simulink model "P_decouple_single_rov"  (Simulink 6.0)
settings: Solver=ode45  StartTime=0.0  StopTime=650  RelTol=1e-3
undefined symbols (not defined in the file): B, DQ, DQL, I, m, M, Ma, MaU, rg, sigbuilder_block, T, W, xb, xg, Xudot, yb, yg, Yvdot, zb, zg, Zwdot
libraries: simulink_extras x8, simulink x7
(part 1 of 2)
settings Model: LastModifiedBy=c chin

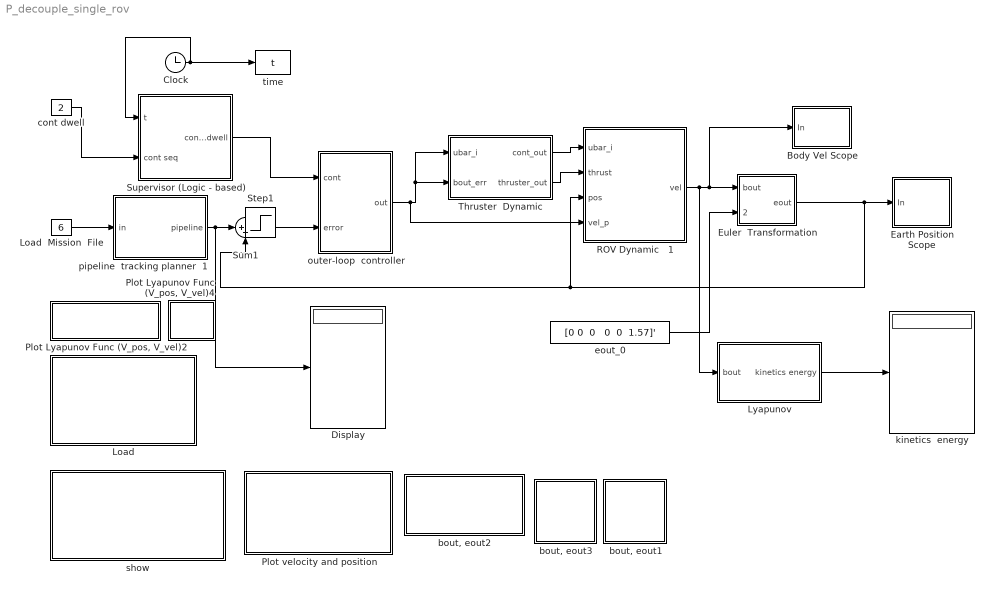
== system P_decouple_single_rov ==
  " Load  " : Subsystem  AncestorBlock=|
      | rov_design_analysis/ROV Controller
      | Design
      | Applications/ Load RRCROV2 parameters
      settings: OpenFcn=|
      | clc
      | cd c:\Matlab7\toolbox\rov_design_analysis\\mat_file ;
      | load rrcrovf;
      mask Display: disp('Double-click \n to \n Load the\n RRCROV\n parameters')
  " ROV Dynamic   1" : Subsystem
      mask Display:
      | disp('ROV')
      | image(imread('/rov_design_analysis/fig/ROVRRC2.jpg'));
      | color('white');port_label('input',1,'ubar_i')
      | color('white');port_label('input',2,'thrust')
      | color('white');port_label('input',3,'eout')
      | color('white');port_label('input',4,'bout_p')
      | 
      | color('white');port_label('output',1,'vel')
  Body Vel Scope : Subsystem  AncestorBlock=|
      | rov_design_analysis/ROV Controller
      | Design
      | Applications/1. Heading autopilot/Earth Position
      | Scope
      mask Display: disp('Body\nVelocity\nScope')
  Clock : Clock
      settings: Decimation=10
  Display : Display
  "Earth Position Scope " : Subsystem  AncestorBlock=|
      | rov_design_analysis/ROV Controller
      | Design
      | Applications/1. Heading autopilot/Earth Position
      | Scope
      mask Display: disp('Earth\nPosition\nScope')
  Euler  Transformation : Subsystem  AncestorBlock=rov_design_analysis/Scope Utilities/Euler Transformation
      mask Display: disp('Navigation \n Sensor')
  Load  Mission  File : Constant  Value=6
  Lyapunov : Subsystem  AncestorBlock=|
      | rov_design_analysis/ROV Controller
      | Design
      | Applications/1. Heading autopilot/pipe tracking
      | profile
      | (Auto)
  "Plot Lyapunov Func (V_pos, V_vel)2" : Subsystem  AncestorBlock=|
      | rov_design_analysis/ROV Controller
      | Design
      | Applications/Plot velocity and position
      settings: OpenFcn=|
      | clc
      | close all
      mask Display: disp('Close All Figure')
  "Plot Lyapunov Func (V_pos, V_vel)4" : Subsystem  AncestorBlock=|
      | rov_design_analysis/ROV Controller
      | Design
      | Applications/Plot velocity and position
      settings: OpenFcn=|
      | clc
      | clear
      mask Display: disp('Clear')
  Plot velocity and position : Subsystem  AncestorBlock=|
      | rov_design_analysis/ROV Controller
      | Design
      | Applications/Plot velocity and position
      settings: OpenFcn=|
      | clc
      | cd c:\Matlab7\toolbox\rov_design_analysis\\m_file ;
      | run nonlin_resp6
      mask Display: disp('Double-click \n to \n Plot Velocity \n and \n Position')
  Sum1 : Sum  Inputs=|+-  OutDataTypeMode=double  SaturateOnIntegerOverflow=on
  Supervisor (Logic - based) : Subsystem
      mask Display: disp('Supervisor \n (Logic-based)')
  Thruster  Dynamic : Subsystem
      mask Display: disp('Thruster \n Dynamic')
  "bout, eout1" : Subsystem  AncestorBlock=|
      | rov_design_analysis/ROV Controller
      | Design
      | Applications/Plot velocity and position
      settings: OpenFcn=|
      | clc
      | cd c:\Matlab7\toolbox\rov_design_analysis\\m_file ;
      | figure
      | plot(eout(:,1),-eout(:,3))
      | xlabel('x')
      | ylabel('z')
      mask Display: disp('Plot \n XZ ')
  "bout, eout2" : Subsystem  AncestorBlock=|
      | rov_design_analysis/ROV Controller
      | Design
      | Applications/Plot velocity and position
      settings: OpenFcn=|
      | clc
      | cd c:\Matlab7\toolbox\rov_design_analysis\\m_file ;
      | figure
      | plot3(eout(:,1), eout(:,2),-eout(:,3))
      | xlabel('x')
      | ylabel('y')
      | zlabel('z')
      | grid on
      mask Display: disp('Plot \n 3D Response')
  "bout, eout3" : Subsystem  AncestorBlock=|
      | rov_design_analysis/ROV Controller
      | Design
      | Applications/Plot velocity and position
      settings: OpenFcn=|
      | clc
      | cd c:\Matlab7\toolbox\rov_design_analysis\\m_file ;
      | figure
      | plot(eout(:,1), eout(:,2))
      | xlabel('x')
      | ylabel('y')
      mask Display: disp('Plot \n XY ')
  cont dwell : Constant  Value=2
  eout_0 : Constant  Value="[0 0  0   0  0  1.57]'"  OutDataTypeMode=double
  kinetics  energy : Display
  outer-loop  controller : Subsystem  Description=f(x)  AncestorBlock=|
      | rov_design_analysis/ROV Controller
      | Design
      | Applications/1. Heading autopilot/controller
      mask Display: disp('Outer Loop \n Controller')
  pipeline  tracking planner  1 : Subsystem  AncestorBlock=|
      | rov_design_analysis/ROV Controller
      | Design
      | Applications/1. Heading autopilot/pipe tracking
      | profile
      | (Auto)
      mask Display: disp('Pipeline Tracking \n Planner')
  show : Subsystem  AncestorBlock=|
      | rov_design_analysis/ROV Controller
      | Design
      | Applications/ Load RRCROV2 parameters
      settings: OpenFcn=|
      | clc
      | cd  c:\Matlab7\toolbox\rov_design_analysis\hybrid ;
      | open rrcrov2_para
      mask Display: disp('Double-click \n to \n SHOW\n RRCROV\n parameters')
  time : ToWorkspace  VariableName=t  SampleTime=1  SaveFormat=Array
  Step1 : Step  IOType=siggen  SampleTime=0
  wires:
  " ROV Dynamic   1"/1(vel) -> Euler  Transformation/1(bout), Body Vel Scope/1(In), Lyapunov/1(bout)
  Euler  Transformation/1(eout) -> "Earth Position Scope "/1(In), Sum1/2, " ROV Dynamic   1"/3("pos ")
  Clock/1 -> time/1, Supervisor (Logic - based)/1(t)
  pipeline  tracking planner  1/1(pipeline) -> Sum1/1, Display/1
  Supervisor (Logic - based)/1(cont dwell) -> outer-loop  controller/1(cont)
  cont dwell/1 -> Supervisor (Logic - based)/2(cont seq)
  eout_0/1 -> Euler  Transformation/2(eout_0)
  Sum1/1 -> outer-loop  controller/2(error)
  Load  Mission  File/1 -> pipeline  tracking planner  1/1(in)
  Thruster  Dynamic/1(cont_out) -> " ROV Dynamic   1"/1(ubar_i)
  Thruster  Dynamic/2(thruster_out) -> " ROV Dynamic   1"/2("thrust ")
  Lyapunov/1(kinetics energy) -> kinetics  energy/1
  outer-loop  controller/1(out) -> Thruster  Dynamic/2(bout_err), Thruster  Dynamic/1(ubar_i), " ROV Dynamic   1"/4(vel_p)

== system P_decouple_single_rov/ Load   ==

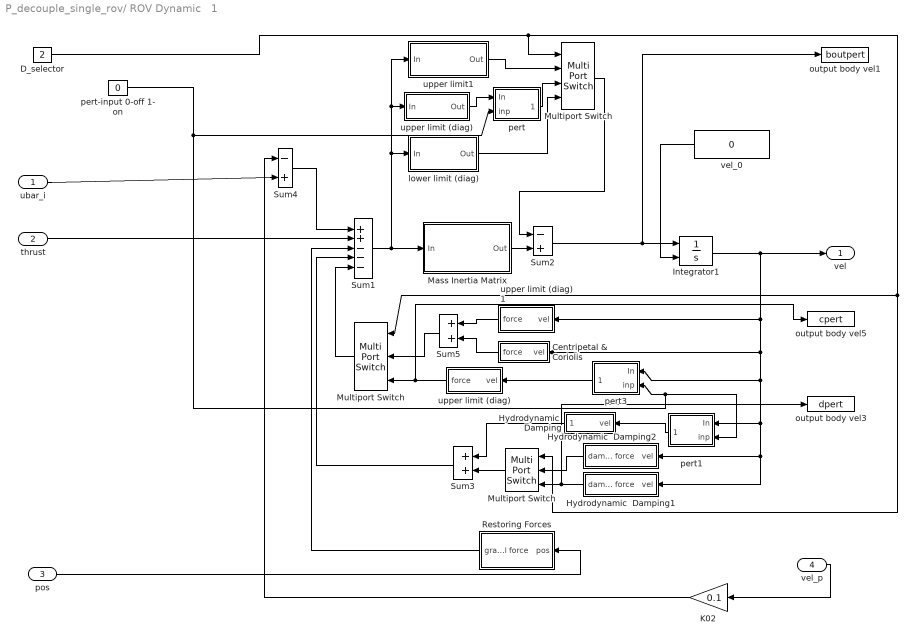
== system P_decouple_single_rov/ ROV Dynamic   1 ==
  ubar_i : Inport  Port=1  LatchInput=off
  "thrust " : Inport  Port=2  LatchInput=off
  "pos " : Inport  Port=3  LatchInput=off
  vel_p : Inport  Port=4  LatchInput=off
  Centripetal & Coriolis : Subsystem  Orientation=left  AncestorBlock=rov_design_analysis/ROV Models/1. Six DOF RRC ROV II/Centripetal & Coriolis
      mask Display: disp('C')
  D_selector : Constant  Value=2
  Hydrodynamic  Damping : Subsystem  Orientation=left
      mask Display: disp('D')
  Hydrodynamic  Damping1 : Subsystem  Orientation=left
      mask Display: disp('perturb \nDamping')
  Hydrodynamic  Damping2 : Subsystem  Orientation=left
      mask Display: disp('Zero Perturb')
  Integrator1 : Integrator  InitialConditionSource=external
  K02 : Gain  Orientation=left  Gain=0.1  SaturateOnIntegerOverflow=on
  Mass Inertia Matrix : Subsystem
      mask Display: disp('inv(MRB+MA)')
  Multiport Switch : MultiPortSwitch  Inputs=3
  "Multiport Switch  " : MultiPortSwitch  Orientation=left  Inputs=2
  "Multiport Switch    " : MultiPortSwitch  Orientation=left  Inputs=2
  Restoring Forces : Subsystem  Orientation=left
      mask Display: disp('Restoring\nForce')
  Sum1 : Sum  Inputs=++---  SaturateOnIntegerOverflow=on  InputSameDT=on
  Sum2 : Sum  Inputs=-+  SaturateOnIntegerOverflow=on  InputSameDT=on
  Sum3 : Sum  Orientation=left  SaturateOnIntegerOverflow=on  InputSameDT=on
  Sum4 : Sum  Inputs=|-+  SaturateOnIntegerOverflow=on  InputSameDT=on
  Sum5 : Sum  Orientation=left  SaturateOnIntegerOverflow=on  InputSameDT=on
  lower limit (diag) : Subsystem
      mask Display: disp('Perturb MA')
  output body vel1 : ToWorkspace  VariableName=boutpert  SampleTime=1  SaveFormat=Array
  output body vel3 : ToWorkspace  VariableName=dpert  SampleTime=1  SaveFormat=Array
  output body vel5 : ToWorkspace  VariableName=cpert  SampleTime=1  SaveFormat=Array
  pert : Subsystem
  pert-input 0-off 1- on : Constant  Value=0
  pert1 : Subsystem  Orientation=left
  pert3 : Subsystem  Orientation=left
  upper limit (diag) : Subsystem
      mask Display: disp('Perturb MA')
  "upper limit (diag)   " : Subsystem  Orientation=left
      mask Display: disp('Perturb CA')
  upper limit (diag)   1 : Subsystem  Orientation=left
      mask Display: disp('CA')
  upper limit1 : Subsystem
      mask Display: disp('Zero Perturb')
  vel_0 : Constant  Orientation=left  Value=0  OutDataTypeMode=double
  vel : Outport
  wires:
  Restoring Forces/1(gravitational force) -> Sum1/3
  "thrust "/1 -> Sum1/2
  Sum1/1 -> Mass Inertia Matrix/1(In), upper limit1/1(In), upper limit (diag)/1(In), lower limit (diag)/1(In)
  "Multiport Switch  "/1 -> Sum1/5
  "pos "/1 -> Restoring Forces/1(pos)
  Mass Inertia Matrix/1(Out) -> Sum2/2
  upper limit1/1(Out) -> Multiport Switch/2
  lower limit (diag)/1(Out) -> Multiport Switch/4
  Multiport Switch/1 -> Sum2/1
  "upper limit (diag)   "/1(force) -> "Multiport Switch  "/3, output body vel5/1
  Sum5/1 -> "Multiport Switch  "/2
  Hydrodynamic  Damping1/1(damping force) -> "Multiport Switch    "/3, output body vel3/1
  Hydrodynamic  Damping2/1(damping force) -> "Multiport Switch    "/2
  Sum3/1 -> Sum1/4
  "Multiport Switch    "/1 -> Sum3/2
  Hydrodynamic  Damping/1(damping force) -> Sum3/1
  upper limit (diag)   1/1(force) -> Sum5/1
  Centripetal & Coriolis/1(force) -> Sum5/2
  Sum2/1 -> output body vel1/1, Integrator1/1
  Integrator1/1 -> vel/1, upper limit (diag)   1/1(vel), Centripetal & Coriolis/1(vel), Hydrodynamic  Damping1/1(vel), Hydrodynamic  Damping2/1(vel), pert1/1(In), pert3/1(In)
  vel_0/1 -> Integrator1/2
  K02/1 -> Sum4/1
  ubar_i/1 -> Sum4/2
  Sum4/1 -> Sum1/1
  vel_p/1 -> K02/1
  pert1/1(on/off) -> Hydrodynamic  Damping/1(vel)
  pert3/1(on/off) -> "upper limit (diag)   "/1(vel)
  upper limit (diag)/1(Out) -> pert/1(In)
  pert/1(on/off) -> Multiport Switch/3
  pert-input 0-off 1- on/1 -> pert/2(inp), pert3/2(inp), pert1/2(inp)
  D_selector/1 -> Multiport Switch/1, "Multiport Switch  "/1, "Multiport Switch    "/1

== system P_decouple_single_rov/Body Vel Scope ==
  In : Inport  Port=1  LatchInput=off
  Demux : Demux  Outputs=6
  output body vel4 : ToWorkspace  VariableName=bout  SampleTime=1  SaveFormat=Array
  phi : Scope
      settings: TickLabels=on  YMin=-0.125  YMax=0.2  DataFormat=Array
  theta : Scope
      settings: TickLabels=on  TimeRange=200  YMin=-0.05  YMax=0.15  DataFormat=Array
  x : Scope
      settings: TickLabels=on  TimeRange=50  YMin=-0.025  YMax=0.375  DataFormat=Array
  y : Scope
      settings: TickLabels=on  YMin=-0.02  YMax=0.1  DataFormat=Array
  yaw : Scope
      settings: TickLabels=on  TimeRange=200  YMin=-0.05  YMax=0.15  SaveName=ScopeData2  DataFormat=Array
  z : Scope
      settings: TickLabels=on  TimeRange=50  YMin=-0.0025  YMax=0.0375  DataFormat=Array
  wires:
  Demux/5 -> theta/1
  In/1 -> Demux/1, output body vel4/1
  Demux/3 -> z/1
  Demux/4 -> phi/1
  Demux/2 -> y/1
  Demux/1 -> x/1
  Demux/6 -> yaw/1

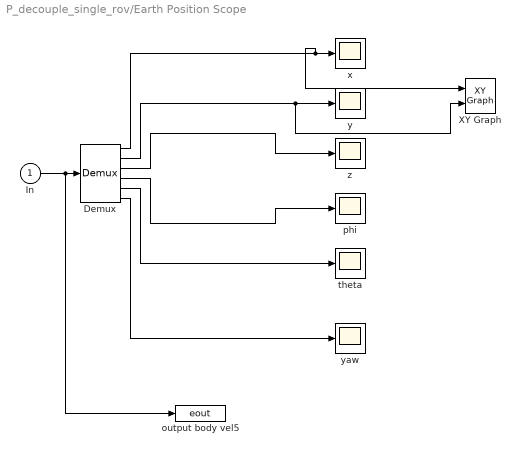
== system P_decouple_single_rov/Earth Position Scope  ==
  In : Inport  Port=1  LatchInput=off
  Demux : Demux  Outputs=6
  XY Graph : simulink/Sinks/XY Graph  xmin=-50  xmax=50  ymin=-50  ymax=50  st=-1
  output body vel5 : ToWorkspace  VariableName=eout  SampleTime=1  SaveFormat=Array
  phi : Scope
      settings: TickLabels=on  YMin=-0.125  YMax=0.2  DataFormat=Array
  theta : Scope
      settings: TickLabels=on  TimeRange=200  YMin=-0.05  YMax=0.15  DataFormat=Array
  x : Scope
      settings: TickLabels=on  TimeRange=50  YMin=-0.025  YMax=0.375  DataFormat=Array
  y : Scope
      settings: TickLabels=on  YMin=-0.02  YMax=0.1  DataFormat=Array
  yaw : Scope
      settings: TickLabels=on  TimeRange=200  YMin=-0.05  YMax=0.15  SaveName=ScopeData2  DataFormat=Array
  z : Scope
      settings: TickLabels=on  TimeRange=50  YMin=-0.0025  YMax=0.0375  DataFormat=Array
  wires:
  Demux/5 -> theta/1
  In/1 -> Demux/1, output body vel5/1
  Demux/3 -> z/1
  Demux/4 -> phi/1
  Demux/2 -> y/1, XY Graph/2
  Demux/1 -> x/1, XY Graph/1
  Demux/6 -> yaw/1

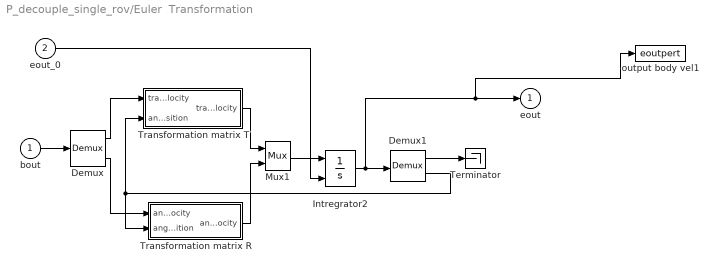
== system P_decouple_single_rov/Euler  Transformation ==
  bout : Inport  Port=1  LatchInput=off
  eout_0 : Inport  Port=2  LatchInput=off
  Demux : Demux  Outputs=2
  Demux1 : Demux  Outputs=2
  Intregrator2 : Integrator  InitialConditionSource=external
  Mux1 : Mux  Inputs=2
  Terminator : Terminator
  Transformation matrix R : Subsystem
      mask Display: disp('Transformation R')
  Transformation matrix T : Subsystem
      mask Display: disp('Transformation T')
  output body vel1 : ToWorkspace  VariableName=eoutpert  SampleTime=1  SaveFormat=Array
  eout : Outport  InitialOutput=0
  wires:
  Mux1/1 -> Intregrator2/1
  Intregrator2/1 -> Demux1/1, eout/1, output body vel1/1
  Demux/2 -> Transformation matrix R/1(angular body  velocity)
  Demux/1 -> Transformation matrix T/1(translational body velocity)
  bout/1 -> Demux/1
  Demux1/2 -> Transformation matrix T/2(angular position), Transformation matrix R/2(angular position)
  Transformation matrix R/1(angular earth velocity) -> Mux1/2
  Transformation matrix T/1(translational earth velocity) -> Mux1/1
  Demux1/1 -> Terminator/1
  eout_0/1 -> Intregrator2/2

== system P_decouple_single_rov/Lyapunov ==
  bout : Inport  Port=1  LatchInput=off
  Gain : Gain  Gain=0.5
  Mass Inertia Matrix1 : Subsystem
      mask Display: disp('MRB+MA')
  Math Function1 : Math  Operator=square  SaturateOnIntegerOverflow=on
  kinetics energy : Outport
  wires:
  Math Function1/1 -> Mass Inertia Matrix1/1(In)
  Gain/1 -> Math Function1/1
  bout/1 -> Gain/1
  Mass Inertia Matrix1/1(Out) -> kinetics energy/1

== system P_decouple_single_rov/Plot Lyapunov Func (V_pos, V_vel)2 ==

== system P_decouple_single_rov/Plot Lyapunov Func (V_pos, V_vel)4 ==

== system P_decouple_single_rov/Plot velocity and position ==

== system P_decouple_single_rov/Supervisor (Logic - based) ==
  t : Inport  Port=1  LatchInput=off
  cont seq : Inport  Port=2  LatchInput=off
  150-300 : Relay  OnSwitchValue=150  OffSwitchValue=0  OnOutputValue=0  OffOutputValue=1
  Constant1 : Constant
  Switching sequence : Subsystem  AncestorBlock=rov_design_analysis/Scope Utilities/Switching sequence
      mask Display: disp('Dwell \n Sequence')
  "cont dwell switch  " : MultiPortSwitch  Inputs=3
  cont dwell : Outport
  wires:
  cont seq/1 -> "cont dwell switch  "/1
  "cont dwell switch  "/1 -> cont dwell/1
  t/1 -> 150-300/1
  Constant1/1 -> "cont dwell switch  "/2
  150-300/1 -> "cont dwell switch  "/3  "1"
  Switching sequence/1(" ") -> "cont dwell switch  "/4  "3"

== system P_decouple_single_rov/Thruster  Dynamic ==
  ubar_i : Inport  Port=1  LatchInput=off
  bout_err : Inport  Port=2  LatchInput=off
  Thruster configuration1 : Subsystem  AncestorBlock=|
      | rov_design_analysis/ROV Controller
      | Design
      | Applications/1. Heading autopilot/Thruster
      | configuration
      mask Display: disp('T')
  Thruster configuration4 : Subsystem  AncestorBlock=|
      | rov_design_analysis/ROV Controller
      | Design
      | Applications/1. Heading autopilot/Thruster
      | configuration
      mask Display: disp('T')
  thruster  dynamic     1 : Subsystem
  thruster  dynamic     2 : Subsystem
  cont_out : Outport
  thruster_out : Outport  Port=2
  wires:
  Thruster configuration1/1(output force) -> thruster_out/1
  thruster  dynamic     1/1(T) -> Thruster configuration4/1(input velocity)
  Thruster configuration4/1(output force) -> cont_out/1
  thruster  dynamic     2/1(T) -> Thruster configuration1/1(input velocity)
  bout_err/1 -> thruster  dynamic     2/1(volt)
  ubar_i/1 -> thruster  dynamic     1/1(volt)

== system P_decouple_single_rov/bout, eout1 ==

== system P_decouple_single_rov/bout, eout2 ==

== system P_decouple_single_rov/bout, eout3 ==

== system P_decouple_single_rov/outer-loop  controller ==
  cont : Inport  Port=1  LatchInput=off
  error : Inport  Port=2  LatchInput=off
  Multiport Switch : MultiPortSwitch  Inputs=2
  "P decoupled " : Subsystem
  PI : Subsystem
  bout input : Constant  Value="[ 0 0  0  0  0 0]'"
  out : Outport
  wires:
  cont/1 -> Multiport Switch/1
  bout input/1 -> "P decoupled "/2(vel_d), "P decoupled "/3(vel)
  Multiport Switch/1 -> out/1
  "P decoupled "/1(" ") -> Multiport Switch/2
  PI/1(" ") -> Multiport Switch/3
  error/1 -> "P decoupled "/1(err), PI/1(err)

== system P_decouple_single_rov/pipeline  tracking planner  1 ==
  in : Inport  Port=1  LatchInput=off
  decoupled input : Subsystem
  pipeline : Outport
  wires:
  in/1 -> decoupled input/1(In1)
  decoupled input/1(Out1) -> pipeline/1

== system P_decouple_single_rov/show ==

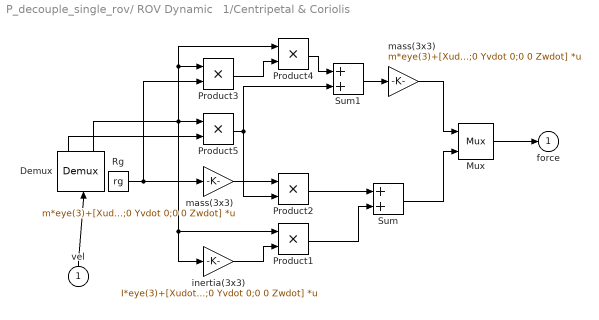
== system P_decouple_single_rov/ ROV Dynamic   1/Centripetal & Coriolis ==
  vel : Inport  Orientation=up  Port=1  LatchInput=off
  Demux : Demux  Orientation=up  Outputs=2
  Mux : Mux  Inputs=2
  Product{1..5} (5 alike) : Product  SaturateOnIntegerOverflow=on  RndMeth=Zero  InputSameDT=on
  Rg : Constant  Value=rg
  Sum : Sum  SaturateOnIntegerOverflow=on  InputSameDT=on
  Sum1 : Sum  SaturateOnIntegerOverflow=on  InputSameDT=on
  inertia(3x3) : Gain  Gain=I*eye(3)+[Xudot 0 0;0 Yvdot 0;0 0 Zwdot]  Multiplication=Matrix(K*u)  SaturateOnIntegerOverflow=on
  "mass(3x3) " : Gain  Gain=m*eye(3)+[Xudot 0 0;0 Yvdot 0;0 0 Zwdot]  Multiplication=Matrix(K*u)  SaturateOnIntegerOverflow=on
  "mass(3x3)   " : Gain  Gain=m*eye(3)+[Xudot 0 0;0 Yvdot 0;0 0 Zwdot]  Multiplication=Matrix(K*u)  SaturateOnIntegerOverflow=on
  force : Outport  InitialOutput=0
  wires:
  Product1/1 -> Sum/2
  "mass(3x3)   "/1 -> Product2/1
  Product2/1 -> Sum/1
  Rg/1 -> Product3/2, "mass(3x3)   "/1
  Product3/1 -> Product4/2
  Product4/1 -> Sum1/1
  Product5/1 -> Product2/2, Sum1/2
  Sum1/1 -> "mass(3x3) "/1
  Demux/2 -> Product5/1, Product3/1, Product4/1, Product1/1, inertia(3x3)/1
  Demux/1 -> Product5/2
  vel/1 -> Demux/1
  inertia(3x3)/1 -> Product1/2
  "mass(3x3) "/1 -> Mux/1
  Sum/1 -> Mux/2
  Mux/1 -> force/1

== system P_decouple_single_rov/ ROV Dynamic   1/Hydrodynamic  Damping ==
  vel : Inport  Port=1  LatchInput=off
  D linear : Gain  Gain=-diag(DQL)  SaturateOnIntegerOverflow=on
  damping force : Outport  InitialOutput=0
  wires:
  vel/1 -> D linear/1
  D linear/1 -> damping force/1

== system P_decouple_single_rov/ ROV Dynamic   1/Hydrodynamic  Damping1 ==
  vel : Inport  Port=1  LatchInput=off
  D quadratic : Gain  Gain=-diag(DQ)  SaturateOnIntegerOverflow=on
  Product : Product  SaturateOnIntegerOverflow=on  RndMeth=Zero  InputSameDT=on
  |u| : Abs  SaturateOnIntegerOverflow=on
  damping force : Outport  InitialOutput=0
  wires:
  Product/1 -> D quadratic/1
  vel/1 -> Product/1, |u|/1
  |u|/1 -> Product/2
  D quadratic/1 -> damping force/1

== system P_decouple_single_rov/ ROV Dynamic   1/Hydrodynamic  Damping2 ==
  vel : Inport  Port=1  LatchInput=off
  D quadratic : Gain  Gain=0  SaturateOnIntegerOverflow=on
  damping force : Outport  InitialOutput=0
  wires:
  vel/1 -> D quadratic/1
  D quadratic/1 -> damping force/1

== system P_decouple_single_rov/ ROV Dynamic   1/Mass Inertia Matrix ==
  In : Inport  Port=1  LatchInput=off
  inverse M : Gain  Gain=inv(M-Ma)  Multiplication=Matrix(K*u)  SaturateOnIntegerOverflow=on
  Out : Outport
  wires:
  inverse M/1 -> Out/1
  In/1 -> inverse M/1

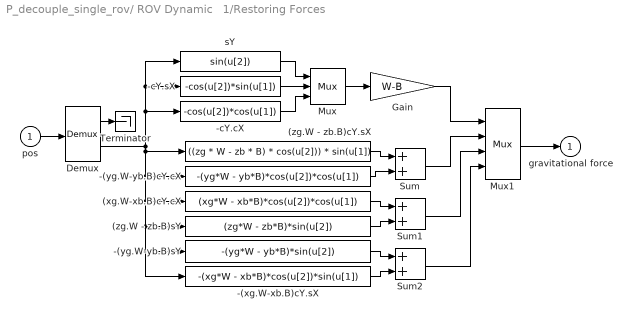
== system P_decouple_single_rov/ ROV Dynamic   1/Restoring Forces ==
  pos : Inport  Port=1  LatchInput=off
  (xg.W-xb.B)cY.cX : Fcn  Expr=(xg*W - xb*B)*cos(u[2])*cos(u[1])
  (zg.W - zb.B)cY.sX : Fcn  Expr=((zg * W - zb * B) * cos(u[2])) * sin(u[1])
  (zg.W - zb.B)sY : Fcn  Expr=(zg*W - zb*B)*sin(u[2])
  -(xg.W-xb.B)cY.sX : Fcn  Expr=-(xg*W - xb*B)*cos(u[2])*sin(u[1])
  -(yg.W-yb.B)cY.cX : Fcn  Expr=-(yg*W - yb*B)*cos(u[2])*cos(u[1])
  -(yg.W-yb.B)sY : Fcn  Expr=-(yg*W - yb*B)*sin(u[2])
  -cY.cX : Fcn  Expr=-cos(u[2])*cos(u[1])
  -cY.sX : Fcn  Expr=-cos(u[2])*sin(u[1])
  Demux : Demux  Outputs=2
  Gain : Gain  Gain=W-B  SaturateOnIntegerOverflow=on
  Mux : Mux  Inputs=3
  Mux1 : Mux
  Sum : Sum  SaturateOnIntegerOverflow=on  InputSameDT=on
  Sum1 : Sum  SaturateOnIntegerOverflow=on  InputSameDT=on
  Sum2 : Sum  SaturateOnIntegerOverflow=on  InputSameDT=on
  Terminator : Terminator
  sY : Fcn  Expr=sin(u[2])
  gravitational force : Outport  InitialOutput=0
  wires:
  Sum2/1 -> Mux1/4
  -(yg.W-yb.B)sY/1 -> Sum2/1
  -(xg.W-xb.B)cY.sX/1 -> Sum2/2
  Sum1/1 -> Mux1/3
  (xg.W-xb.B)cY.cX/1 -> Sum1/1
  (zg.W - zb.B)sY/1 -> Sum1/2
  Sum/1 -> Mux1/2
  (zg.W - zb.B)cY.sX/1 -> Sum/1
  -(yg.W-yb.B)cY.cX/1 -> Sum/2
  Gain/1 -> Mux1/1
  Mux/1 -> Gain/1
  -cY.cX/1 -> Mux/3
  -cY.sX/1 -> Mux/2
  sY/1 -> Mux/1
  Mux1/1 -> gravitational force/1
  Demux/2 -> -(xg.W-xb.B)cY.sX/1, -(yg.W-yb.B)sY/1, (zg.W - zb.B)sY/1, (xg.W-xb.B)cY.cX/1, -(yg.W-yb.B)cY.cX/1, (zg.W - zb.B)cY.sX/1, sY/1, -cY.sX/1, -cY.cX/1
  Demux/1 -> Terminator/1
  pos/1 -> Demux/1

== system P_decouple_single_rov/ ROV Dynamic   1/lower limit (diag) ==
  In : Inport  Port=1  LatchInput=off
  inverse M : Gain  Gain=-diag([21.1403-21.0981 51.7012-51.0026 92.451-91.837 3.6191-3.576 2.6427-2.7687 2.3033-2.3493])  Multiplication=Matrix(K*u)  SaturateOnIntegerOverflow=on
  Out : Outport
  wires:
  inverse M/1 -> Out/1
  In/1 -> inverse M/1

== system P_decouple_single_rov/ ROV Dynamic   1/pert ==
  In : Inport  Port=1  LatchInput=off
  inp : Inport  Port=2  LatchInput=off
  D linear3 : Gain  Gain=2  SaturateOnIntegerOverflow=on
  Product : Product  RndMeth=Zero
  Sine Wave-pert : Sin  Amplitude=0.1  SampleTime=0
  Sum6 : Sum  Inputs=|++  SaturateOnIntegerOverflow=on  InputSameDT=on
  on/off : Outport
  wires:
  D linear3/1 -> Sum6/1
  Sine Wave-pert/1 -> Product/1
  Product/1 -> Sum6/2
  inp/1 -> Product/2
  In/1 -> D linear3/1
  Sum6/1 -> on/off/1

== system P_decouple_single_rov/ ROV Dynamic   1/pert1 ==
  In : Inport  Port=1  LatchInput=off
  inp : Inport  Port=2  LatchInput=off
  D linear3 : Gain  Gain=2  SaturateOnIntegerOverflow=on
  Product : Product  RndMeth=Zero
  Sine Wave-pert : Sin  Amplitude=0.1  SampleTime=0
  Sum6 : Sum  Inputs=|++  SaturateOnIntegerOverflow=on  InputSameDT=on
  on/off : Outport
  wires:
  D linear3/1 -> Sum6/1
  Sine Wave-pert/1 -> Product/1
  Product/1 -> Sum6/2
  inp/1 -> Product/2
  In/1 -> D linear3/1
  Sum6/1 -> on/off/1

== system P_decouple_single_rov/ ROV Dynamic   1/pert3 ==
  In : Inport  Port=1  LatchInput=off
  inp : Inport  Port=2  LatchInput=off
  D linear3 : Gain  Gain=2  SaturateOnIntegerOverflow=on
  Product : Product  RndMeth=Zero
  Sine Wave-pert : Sin  Amplitude=0.1  SampleTime=0
  Sum6 : Sum  Inputs=|++  SaturateOnIntegerOverflow=on  InputSameDT=on
  on/off : Outport
  wires:
  D linear3/1 -> Sum6/1
  Sine Wave-pert/1 -> Product/1
  Product/1 -> Sum6/2
  inp/1 -> Product/2
  In/1 -> D linear3/1
  Sum6/1 -> on/off/1

== system P_decouple_single_rov/ ROV Dynamic   1/upper limit (diag) ==
  In : Inport  Port=1  LatchInput=off
  inverse M : Gain  Gain=-diag([21.724-21.1403 51.7013-51.7012 94.3-92.451 4.2176-3.6191 7.1148-2.6427 4.7673-2.3033])  Multiplication=Matrix(K*u)  SaturateOnIntegerOverflow=on
  Out : Outport
  wires:
  inverse M/1 -> Out/1
  In/1 -> inverse M/1

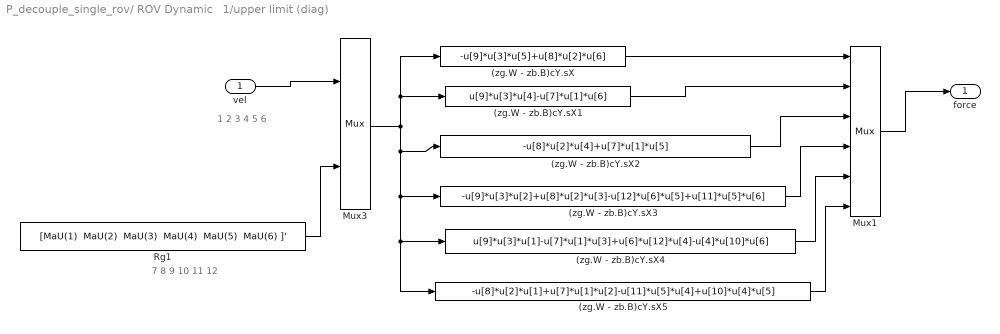
== system P_decouple_single_rov/ ROV Dynamic   1/upper limit (diag)    ==
  note: 7 8 9 10 11 12
  note: 1 2 3 4 5 6
  vel : Inport  Port=1  LatchInput=off
  (zg.W - zb.B)cY.sX : Fcn  Expr=-u[9]*u[3]*u[5]+u[8]*u[2]*u[6]
  (zg.W - zb.B)cY.sX1 : Fcn  Expr=u[9]*u[3]*u[4]-u[7]*u[1]*u[6]
  (zg.W - zb.B)cY.sX2 : Fcn  Expr=-u[8]*u[2]*u[4]+u[7]*u[1]*u[5]
  (zg.W - zb.B)cY.sX3 : Fcn  Expr=-u[9]*u[3]*u[2]+u[8]*u[2]*u[3]-u[12]*u[6]*u[5]+u[11]*u[5]*u[6]
  (zg.W - zb.B)cY.sX4 : Fcn  Expr=u[9]*u[3]*u[1]-u[7]*u[1]*u[3]+u[6]*u[12]*u[4]-u[4]*u[10]*u[6]
  (zg.W - zb.B)cY.sX5 : Fcn  Expr=-u[8]*u[2]*u[1]+u[7]*u[1]*u[2]-u[11]*u[5]*u[4]+u[10]*u[4]*u[5]
  Mux1 : Mux  Inputs=6
  Mux3 : Mux  Inputs=2
  Rg1 : Constant  Value="[MaU(1)  MaU(2)  MaU(3)  MaU(4)  MaU(5)  MaU(6) ]'"
  force : Outport
  wires:
  Mux1/1 -> force/1
  (zg.W - zb.B)cY.sX/1 -> Mux1/1
  (zg.W - zb.B)cY.sX1/1 -> Mux1/2
  (zg.W - zb.B)cY.sX2/1 -> Mux1/3
  (zg.W - zb.B)cY.sX3/1 -> Mux1/4
  (zg.W - zb.B)cY.sX4/1 -> Mux1/5
  (zg.W - zb.B)cY.sX5/1 -> Mux1/6
  vel/1 -> Mux3/1
  Rg1/1 -> Mux3/2
  Mux3/1 -> (zg.W - zb.B)cY.sX/1, (zg.W - zb.B)cY.sX1/1, (zg.W - zb.B)cY.sX4/1, (zg.W - zb.B)cY.sX5/1, (zg.W - zb.B)cY.sX3/1, (zg.W - zb.B)cY.sX2/1

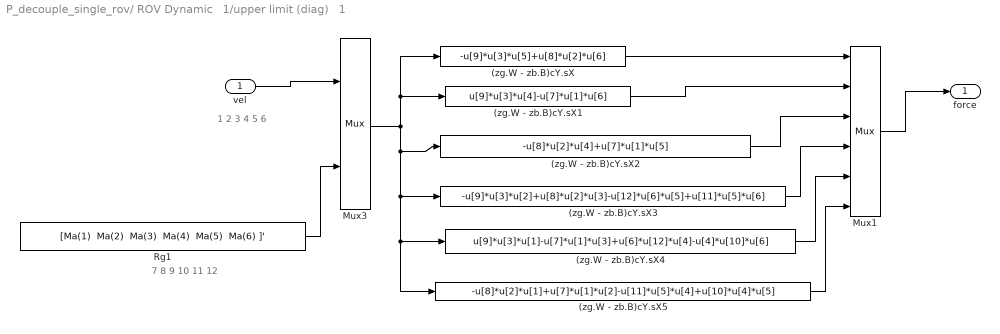
== system P_decouple_single_rov/ ROV Dynamic   1/upper limit (diag)   1 ==
  note: 7 8 9 10 11 12
  note: 1 2 3 4 5 6
  vel : Inport  Port=1  LatchInput=off
  (zg.W - zb.B)cY.sX : Fcn  Expr=-u[9]*u[3]*u[5]+u[8]*u[2]*u[6]
  (zg.W - zb.B)cY.sX1 : Fcn  Expr=u[9]*u[3]*u[4]-u[7]*u[1]*u[6]
  (zg.W - zb.B)cY.sX2 : Fcn  Expr=-u[8]*u[2]*u[4]+u[7]*u[1]*u[5]
  (zg.W - zb.B)cY.sX3 : Fcn  Expr=-u[9]*u[3]*u[2]+u[8]*u[2]*u[3]-u[12]*u[6]*u[5]+u[11]*u[5]*u[6]
  (zg.W - zb.B)cY.sX4 : Fcn  Expr=u[9]*u[3]*u[1]-u[7]*u[1]*u[3]+u[6]*u[12]*u[4]-u[4]*u[10]*u[6]
  (zg.W - zb.B)cY.sX5 : Fcn  Expr=-u[8]*u[2]*u[1]+u[7]*u[1]*u[2]-u[11]*u[5]*u[4]+u[10]*u[4]*u[5]
  Mux1 : Mux  Inputs=6
  Mux3 : Mux  Inputs=2
  Rg1 : Constant  Value="[Ma(1)  Ma(2)  Ma(3)  Ma(4)  Ma(5)  Ma(6) ]'"
  force : Outport
  wires:
  Mux1/1 -> force/1
  (zg.W - zb.B)cY.sX/1 -> Mux1/1
  (zg.W - zb.B)cY.sX1/1 -> Mux1/2
  (zg.W - zb.B)cY.sX2/1 -> Mux1/3
  (zg.W - zb.B)cY.sX3/1 -> Mux1/4
  (zg.W - zb.B)cY.sX4/1 -> Mux1/5
  (zg.W - zb.B)cY.sX5/1 -> Mux1/6
  vel/1 -> Mux3/1
  Rg1/1 -> Mux3/2
  Mux3/1 -> (zg.W - zb.B)cY.sX/1, (zg.W - zb.B)cY.sX1/1, (zg.W - zb.B)cY.sX4/1, (zg.W - zb.B)cY.sX5/1, (zg.W - zb.B)cY.sX3/1, (zg.W - zb.B)cY.sX2/1

== system P_decouple_single_rov/ ROV Dynamic   1/upper limit1 ==
  In : Inport  Port=1  LatchInput=off
  inverse M : Gain  Gain=0  Multiplication=Matrix(K*u)  SaturateOnIntegerOverflow=on
  Out : Outport
  wires:
  inverse M/1 -> Out/1
  In/1 -> inverse M/1

== system P_decouple_single_rov/Euler  Transformation/Transformation matrix R ==
  angular body  velocity : Inport  Port=1  LatchInput=off
  angular position : Inport  Port=2  LatchInput=off
  Mux : Mux  Inputs=3
  Row1 of T : Subsystem
      mask Display: disp('Row 1')
  Row2 of T : Subsystem
      mask Display: disp('Row 2')
  Row3 of T : Subsystem
      mask Display: disp('Row 3')
  angular earth velocity : Outport
  wires:
  angular position/1 -> Row3 of T/2(angular position), Row1 of T/2(angular position), Row2 of T/2(angular position)
  Mux/1 -> angular earth velocity/1
  Row3 of T/1(angular earth velocity (row 3)) -> Mux/3
  Row2 of T/1(angular earth velocity (row 2)) -> Mux/2
  Row1 of T/1(angular earth velocity (row 1)) -> Mux/1
  angular body  velocity/1 -> Row3 of T/1("angular body velocity "), Row2 of T/1("angular body velocity "), Row1 of T/1(angular body  velocity)

== system P_decouple_single_rov/Euler  Transformation/Transformation matrix T ==
  translational body velocity : Inport  Port=1  LatchInput=off
  angular position : Inport  Port=2  LatchInput=off
  Mux : Mux  Inputs=3
  Row1 of R : Subsystem
      mask Display: disp('Row 1')
  Row2 of R : Subsystem
      mask Display: disp('Row 2')
  Row3 of R : Subsystem
      mask Display: disp('Row 3')
  translational earth velocity : Outport  InitialOutput=0
  wires:
  Mux/1 -> translational earth velocity/1
  Row3 of R/1(translational earth velocity (row 3)) -> Mux/3
  Row2 of R/1(translational earth velocity (row 2)) -> Mux/2
  Row1 of R/1(translational earth velocity (row 1)) -> Mux/1
  angular position/1 -> Row3 of R/2(angular position), Row1 of R/2(angular position), Row2 of R/2(angular position)
  translational body velocity/1 -> Row1 of R/1(translational body velocity), Row2 of R/1(translational body velocity), Row3 of R/1(translational body velocity)

== system P_decouple_single_rov/Lyapunov/Mass Inertia Matrix1 ==
  In : Inport  Port=1  LatchInput=off
  inverse M : Gain  Gain=M-Ma  Multiplication=Matrix(K*u)  SaturateOnIntegerOverflow=on
  Out : Outport
  wires:
  inverse M/1 -> Out/1
  In/1 -> inverse M/1

== system P_decouple_single_rov/Supervisor (Logic - based)/Switching sequence ==
  Add2 : Sum  Inputs=+++++++  OutScaling=2^-10
  Signal Builder2 : Subsystem  Tag=STV Subsys  LoadFcn=sigbuilder_block('load');  StartFcn=sigbuilder_block('start');  StopFcn=sigbuilder_block('stop');  ClipboardFcn=sigbuilder_block('clipboard');  mask(Sigbuilder block){}
      mask help: Sigbuilder GUI
      mask init:
      | if ~strcmp(get_param(bdroot(gcbh),'SimulationStatus'),'stopped') tuvar = sigbuilder_block('maskInit'); end
      settings: CopyFcn=sigbuilder_block('copy');  DeleteFcn=sigbuilder_block('delete');  ModelCloseFcn=sigbuilder_block('modelClose');  PreSaveFcn=sigbuilder_block('preSave');  NameChangeFcn=sigbuilder_block('namechange');  OpenFcn=sigbuilder_block('open',[0 19.5 768 499.5 ]);  CloseFcn=sigbuilder_block('close');
      mask Display: plot(0,0,100,100,[10,10,40,40,10],[80,20,20,80,80],[40,10],[50,50], [40,27,10],[65,72,56],[40,25,25,10],[28,28,43,43]);
  " " : Outport
  wires:
  Add2/1 -> " "/1
  Signal Builder2/7(Signal 7) -> Add2/7
  Signal Builder2/6(Signal 6) -> Add2/6
  Signal Builder2/5(Signal 5) -> Add2/5
  Signal Builder2/4(Signal 4) -> Add2/4
  Signal Builder2/3(Signal 3) -> Add2/3
  Signal Builder2/2(Signal 2) -> Add2/2
  Signal Builder2/1(Signal 1) -> Add2/1

== system P_decouple_single_rov/Thruster  Dynamic/Thruster configuration1 ==
  input velocity : Inport  Orientation=up  Port=1  LatchInput=off
  Thruster Matrix : Gain  Gain=T  Multiplication=Matrix(K*u)  SaturateOnIntegerOverflow=on
  output force : Outport  InitialOutput=0
  wires:
  input velocity/1 -> Thruster Matrix/1
  Thruster Matrix/1 -> output force/1

== system P_decouple_single_rov/Thruster  Dynamic/Thruster configuration4 ==
  input velocity : Inport  Orientation=up  Port=1  LatchInput=off
  Thruster Matrix : Gain  Gain=T  Multiplication=Matrix(K*u)  SaturateOnIntegerOverflow=on
  output force : Outport  InitialOutput=0
  wires:
  input velocity/1 -> Thruster Matrix/1
  Thruster Matrix/1 -> output force/1

== system P_decouple_single_rov/Thruster  Dynamic/thruster  dynamic     1 ==
  volt : Inport  Orientation=down  Port=1  LatchInput=off
  Gain2 : Gain  Gain=0.5  SaturateOnIntegerOverflow=on
  Saturation : Saturate  UpperLimit=70  LowerLimit=-70
  "thruster  alloc. " : Subsystem
  T : Outport
  wires:
  volt/1 -> "thruster  alloc. "/1(err)
  "thruster  alloc. "/1(u) -> Gain2/1
  Saturation/1 -> T/1
  Gain2/1 -> Saturation/1

== system P_decouple_single_rov/Thruster  Dynamic/thruster  dynamic     2 ==
  volt : Inport  Orientation=down  Port=1  LatchInput=off
  Gain2 : Gain  Gain=0.5  SaturateOnIntegerOverflow=on
  Saturation : Saturate  UpperLimit=70  LowerLimit=-70
  "thruster  alloc. " : Subsystem
  T : Outport
  wires:
  volt/1 -> "thruster  alloc. "/1(err)
  "thruster  alloc. "/1(u) -> Gain2/1
  Saturation/1 -> T/1
  Gain2/1 -> Saturation/1

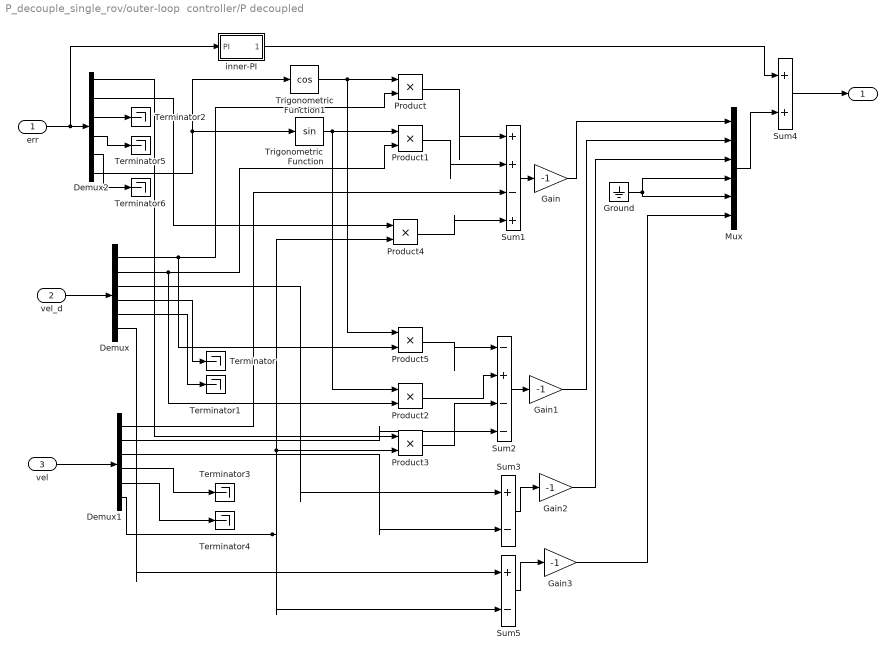
== system P_decouple_single_rov/outer-loop  controller/P decoupled  ==
  err : Inport  Port=1  LatchInput=off
  vel_d : Inport  Port=2  LatchInput=off
  vel : Inport  Port=3  LatchInput=off
  Demux : Demux  Outputs=6
  Demux1 : Demux  Outputs=6
  Demux2 : Demux  Outputs=6
  Gain{,1..3} (4 alike) : Gain  Gain=-1
  Ground : Ground
  Mux : Mux  Inputs=6
  Product{,1..4} (5 alike) : Product  RndMeth=Zero
  Product5 : Product  OutDataTypeMode=double  RndMeth=Zero
  Sum1 : Sum  Inputs=|++-+  SaturateOnIntegerOverflow=on  InputSameDT=on
  Sum2 : Sum  Inputs=|-+--  SaturateOnIntegerOverflow=on  InputSameDT=on
  Sum3 : Sum  Inputs=|+-  SaturateOnIntegerOverflow=on  InputSameDT=on
  Sum4 : Sum  Inputs=|++  SaturateOnIntegerOverflow=on  InputSameDT=on
  Sum5 : Sum  Inputs=|+-  SaturateOnIntegerOverflow=on  InputSameDT=on
  Terminator{,1..6} (7 alike) : Terminator
  Trigonometric Function : Trigonometry
  Trigonometric Function1 : Trigonometry  Operator=cos
  inner-PI : Subsystem
  " " : Outport
  wires:
  err/1 -> Demux2/1, inner-PI/1(PI)
  vel_d/1 -> Demux/1
  Sum2/1 -> Gain1/1
  Sum1/1 -> Gain/1
  Sum3/1 -> Gain2/1
  Ground/1 -> Mux/4, Mux/5
  vel/1 -> Demux1/1
  Demux1/4 -> Terminator3/1
  Demux1/5 -> Terminator4/1
  Trigonometric Function/1 -> Product1/1, Product2/1
  Trigonometric Function1/1 -> Product/1, Product5/1
  Demux2/6 -> Trigonometric Function1/1, Trigonometric Function/1
  Demux/1 -> Product5/2, Product/2
  Demux/2 -> Product2/2, Product1/2
  Product/1 -> Sum1/1
  Product1/1 -> Sum1/2
  Demux1/1 -> Sum1/3
  Product4/1 -> Sum1/4
  Demux1/6 -> Product4/2, Product3/2, Sum5/2
  Demux2/2 -> Product4/1
  Product5/1 -> Sum2/1
  Product2/1 -> Sum2/2
  Product3/1 -> Sum2/3
  Demux2/1 -> Product3/1
  Demux1/2 -> Sum2/4
  Demux/3 -> Sum3/1
  Demux1/3 -> Sum3/2
  Demux/4 -> Terminator/1
  Demux/5 -> Terminator1/1
  Gain/1 -> Mux/1
  Gain1/1 -> Mux/2
  Gain2/1 -> Mux/3
  inner-PI/1(" ") -> Sum4/1
  Mux/1 -> Sum4/2
  Sum4/1 -> " "/1
  Demux2/3 -> Terminator2/1
  Demux2/4 -> Terminator5/1
  Demux2/5 -> Terminator6/1
  Demux/6 -> Sum5/1
  Sum5/1 -> Gain3/1
  Gain3/1 -> Mux/6

== system P_decouple_single_rov/outer-loop  controller/PI ==
  err : Inport  Port=1  LatchInput=off
  Demux1 : Demux  Outputs=6
  Mux2 : Mux  Inputs=6
  P Controller{1..4} (4 alike) : simulink_extras/Additional Linear/PID Controller  P=1  I=1  D=0
  " " : Outport
  wires:
  P Controller3/1 -> Mux2/3
  err/1 -> Demux1/1
  Mux2/1 -> " "/1
  Demux1/1 -> P Controller1/1
  P Controller1/1 -> Mux2/1
  P Controller2/1 -> Mux2/2
  P Controller4/1 -> Mux2/6
  Demux1/2 -> P Controller2/1
  Demux1/3 -> P Controller3/1
  Demux1/6 -> P Controller4/1

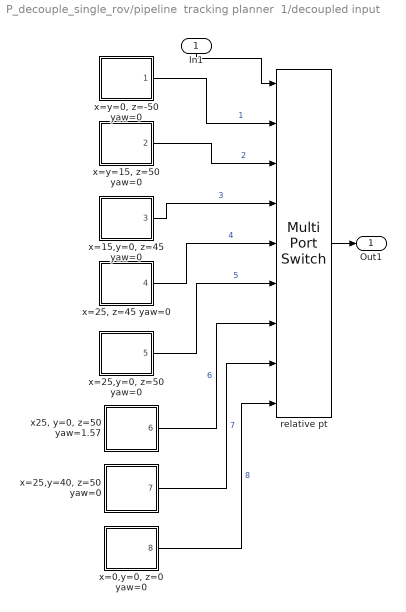
== system P_decouple_single_rov/pipeline  tracking planner  1/decoupled input ==
  In1 : Inport  Orientation=down  Port=1  LatchInput=off
  relative pt : MultiPortSwitch  Inputs=8
  "x25, y=0, z=50 yaw=1.57" : Subsystem
  "x=0,y=0, z=0 yaw=0  " : Subsystem
  "x=15,y=0, z=45 yaw=0 " : Subsystem
  "x=25, z=45 yaw=0" : Subsystem
  "x=25,y=0, z=50 yaw=0" : Subsystem
  "x=25,y=40, z=50 yaw=0" : Subsystem
  "x=y=0, z=-50 yaw=0  " : Subsystem
  "x=y=15, z=50 yaw=0 " : Subsystem
  Out1 : Outport
  wires:
  "x=y=0, z=-50 yaw=0  "/1("1 ") -> relative pt/2  "1"
  "x=y=15, z=50 yaw=0 "/1(2) -> relative pt/3  "2"
  "x=15,y=0, z=45 yaw=0 "/1(3) -> relative pt/4  "3"
  "x=25, z=45 yaw=0"/1(4) -> relative pt/5  "4"
  "x=25,y=0, z=50 yaw=0"/1(5) -> relative pt/6  "5"
  "x25, y=0, z=50 yaw=1.57"/1(6) -> relative pt/7  "6"
  "x=25,y=40, z=50 yaw=0"/1(7) -> relative pt/8  "7"
  "x=0,y=0, z=0 yaw=0  "/1(8) -> relative pt/9  "8"
  In1/1 -> relative pt/1
  relative pt/1 -> Out1/1

== system P_decouple_single_rov/Euler  Transformation/Transformation matrix R/Row1 of T ==
  angular body  velocity : Inport  Port=1  LatchInput=off
  angular position : Inport  Port=2  LatchInput=off
  1 : Fcn  Expr=1
  Dot Product1 : simulink/Math Operations/Dot Product  InputSameDT=on  OutDataType=sfix(16)  OutScaling=2^-10  DoSatur=off
  Mux1 : Mux  Inputs=3
  cX.tY : Fcn  Expr=cos(u[1])*tan(u[2])
  sX.tY : Fcn  Expr=sin(u[1])*tan(u[2])
  angular earth velocity (row 1) : Outport
  wires:
  Dot Product1/1 -> angular earth velocity (row 1)/1
  angular body  velocity/1 -> Dot Product1/2
  Mux1/1 -> Dot Product1/1
  cX.tY/1 -> Mux1/3
  sX.tY/1 -> Mux1/2
  1/1 -> Mux1/1
  angular position/1 -> cX.tY/1, sX.tY/1, 1/1

== system P_decouple_single_rov/Euler  Transformation/Transformation matrix R/Row2 of T ==
  "angular body velocity " : Inport  Port=1  LatchInput=off
  angular position : Inport  Port=2  LatchInput=off
  -sX : Fcn  Expr=-sin(u[1])
  0 : Fcn  Expr=0
  Dot Product1 : simulink/Math Operations/Dot Product  InputSameDT=on  OutDataType=sfix(16)  OutScaling=2^-10  DoSatur=off
  Mux1 : Mux  Inputs=3
  cX : Fcn  Expr=cos(u[1])
  angular earth velocity (row 2) : Outport
  wires:
  Dot Product1/1 -> angular earth velocity (row 2)/1
  "angular body velocity "/1 -> Dot Product1/2
  Mux1/1 -> Dot Product1/1
  -sX/1 -> Mux1/3
  cX/1 -> Mux1/2
  0/1 -> Mux1/1
  angular position/1 -> -sX/1, cX/1, 0/1

== system P_decouple_single_rov/Euler  Transformation/Transformation matrix R/Row3 of T ==
  "angular body velocity " : Inport  Port=1  LatchInput=off
  angular position : Inport  Port=2  LatchInput=off
  1 : Fcn  Expr=0
  Dot Product1 : simulink/Math Operations/Dot Product  InputSameDT=on  OutDataType=sfix(16)  OutScaling=2^-10  DoSatur=off
  Mux1 : Mux  Inputs=3
  cX/cY : Fcn  Expr=cos(u[1])/cos(u[2])
  sX/cY : Fcn  Expr=sin(u[1])/cos(u[2])
  angular earth velocity (row 3) : Outport
  wires:
  Dot Product1/1 -> angular earth velocity (row 3)/1
  "angular body velocity "/1 -> Dot Product1/2
  Mux1/1 -> Dot Product1/1
  cX/cY/1 -> Mux1/3
  sX/cY/1 -> Mux1/2
  1/1 -> Mux1/1
  angular position/1 -> cX/cY/1, sX/cY/1, 1/1

== system P_decouple_single_rov/Euler  Transformation/Transformation matrix T/Row1 of R ==
  translational body velocity : Inport  Port=1  LatchInput=off
  angular position : Inport  Port=2  LatchInput=off
  -sZ.cX+cZ.sY.sX : Fcn  Expr=-sin(u[3])*cos(u[1]) + cos(u[3])*sin(u[2])*sin(u[1])
  Dot Product : simulink/Math Operations/Dot Product  InputSameDT=on  OutDataType=sfix(16)  OutScaling=2^-10  DoSatur=off
  Mux : Mux  Inputs=3
  cY.cZ : Fcn  Expr=cos(u[3]) * cos(u[2])
  sZ.sX+cZ.cX.sY : Fcn  Expr=sin(u[3])*sin(u[1]) + cos(u[3])*cos(u[1])*sin(u[2])
  translational earth velocity (row 1) : Outport
  wires:
  Dot Product/1 -> translational earth velocity (row 1)/1
  translational body velocity/1 -> Dot Product/2
  Mux/1 -> Dot Product/1
  sZ.sX+cZ.cX.sY/1 -> Mux/3
  -sZ.cX+cZ.sY.sX/1 -> Mux/2
  cY.cZ/1 -> Mux/1
  angular position/1 -> sZ.sX+cZ.cX.sY/1, -sZ.cX+cZ.sY.sX/1, cY.cZ/1

== system P_decouple_single_rov/Euler  Transformation/Transformation matrix T/Row2 of R ==
  translational body velocity : Inport  Port=1  LatchInput=off
  angular position : Inport  Port=2  LatchInput=off
  -cZ.sX+sY.sZ.cX : Fcn  Expr=-cos(u[3])*sin(u[1]) + sin(u[2])*sin(u[3])*cos(u[1])
  Dot Product1 : simulink/Math Operations/Dot Product  InputSameDT=on  OutDataType=sfix(16)  OutScaling=2^-10  DoSatur=off
  Mux1 : Mux  Inputs=3
  cY.sZ : Fcn  Expr=sin(u[3]) * cos(u[2])
  cZ.cX+sX.sY.sZ : Fcn  Expr=cos(u[3])*cos(u[1]) + sin(u[1])*sin(u[2])*sin(u[3])
  translational earth velocity (row 2) : Outport
  wires:
  Dot Product1/1 -> translational earth velocity (row 2)/1
  translational body velocity/1 -> Dot Product1/2
  Mux1/1 -> Dot Product1/1
  -cZ.sX+sY.sZ.cX/1 -> Mux1/3
  cZ.cX+sX.sY.sZ/1 -> Mux1/2
  cY.sZ/1 -> Mux1/1
  angular position/1 -> -cZ.sX+sY.sZ.cX/1, cZ.cX+sX.sY.sZ/1, cY.sZ/1

== system P_decouple_single_rov/Euler  Transformation/Transformation matrix T/Row3 of R ==
  translational body velocity : Inport  Port=1  LatchInput=off
  angular position : Inport  Port=2  LatchInput=off
  -sY : Fcn  Expr=-sin(u[2])
  Dot Product1 : simulink/Math Operations/Dot Product  InputSameDT=on  OutDataType=sfix(16)  OutScaling=2^-10  DoSatur=off
  Mux1 : Mux  Inputs=3
  cY.cX : Fcn  Expr=cos(u[2])*cos(u[1])
  cY.sX : Fcn  Expr=cos(u[2])*sin(u[1])
  translational earth velocity (row 3) : Outport  InitialOutput=0
  wires:
  Dot Product1/1 -> translational earth velocity (row 3)/1
  translational body velocity/1 -> Dot Product1/2
  Mux1/1 -> Dot Product1/1
  cY.cX/1 -> Mux1/3
  cY.sX/1 -> Mux1/2
  -sY/1 -> Mux1/1
  angular position/1 -> cY.cX/1, cY.sX/1, -sY/1

== system P_decouple_single_rov/Supervisor (Logic - based)/Switching sequence/Signal Builder2 ==
  Demux : Demux  Tag=STV Demux  Outputs=7
  FromWs : FromWorkspace  Tag=STV FromWs  VariableName=tuvar  SampleTime=0  SigBuilderData=DataTag0  VnvData=DataTag1
      SigBuilderData=|
      | channels(1).label = 'Signal 1'
      | channels(1).allXData = {[0 65 65 700]}
      | channels(1).allYData = {[1 1 0 0]}
      | channels(2).label = 'Signal 2'
      | channels(2).allXData = {[0 70 70 150 150 700]}
      | channels(2).allYData = {[0 0 1 1 0 0]}
      | channels(3).label = 'Signal 3'
      | channels(3).allXData = {[0 160 160 230 230 700]}
      | channels(3).allYData = {[0 0 1 1 0 0]}
      | channels(4).label = 'Signal 4'
      | channels(4).allXData = {[0 240 240 290 290 700]}
      | channels(4).allYData = {[0 0 1 1 0 0]}
      | channels(5).label = 'Signal 5'
      | channels(5).allXData = {[0 300 300 350 350 700]}
      | channels(5).allYData = {[0 0 1 1 0 0]}
      | channels(6).label = 'Signal 6'
      | channels(6).allXData = {[0 360 360 400 400 700]}
      | channels(6).allYData = {[0 0 1 1 0 0]}
      | channels(7).label = 'Signal 7'
      | channels(7).allXData = {[0 410 410 548 548 700]}
      | channels(7).allYData = {[0 0 1 1 0 0]}
      | dataSet.timeRange = [0 700]
      | dataSet.name = 'Group 1'
  Signal 1 : Outport  Tag=STV Outport
  Signal 2 : Outport  Tag=STV Outport  Port=2
  Signal 3 : Outport  Tag=STV Outport  Port=3
  Signal 4 : Outport  Tag=STV Outport  Port=4
  Signal 5 : Outport  Tag=STV Outport  Port=5
  Signal 6 : Outport  Tag=STV Outport  Port=6
  Signal 7 : Outport  Tag=STV Outport  Port=7
  wires:
  Demux/7 -> Signal 7/1
  Demux/6 -> Signal 6/1
  Demux/5 -> Signal 5/1
  Demux/4 -> Signal 4/1
  Demux/3 -> Signal 3/1
  Demux/2 -> Signal 2/1
  FromWs/1 -> Demux/1
  Demux/1 -> Signal 1/1

== system P_decouple_single_rov/Thruster  Dynamic/thruster  dynamic     1/thruster  alloc.  ==
  err : Inport  Port=1  LatchInput=off
  " input" : Constant  Value=[ 1 1 1 1]'
  Selector : Selector  Elements=[1 2 3 6]  InputPortWidth=6
  thruster  allocation control1 : Subsystem  AncestorBlock=|
      | rov_design_analysis/ROV Controller
      | Design
      | Applications/1. Heading autopilot/thruster 
      | allocation control
  u : Outport
  wires:
  err/1 -> Selector/1
  Selector/1 -> thruster  allocation control1/1(vel)
  " input"/1 -> thruster  allocation control1/2(on/off)
  thruster  allocation control1/1(volt) -> u/1

== system P_decouple_single_rov/Thruster  Dynamic/thruster  dynamic     2/thruster  alloc.  ==
  err : Inport  Port=1  LatchInput=off
  " input" : Constant  Value=[ 1 1 1 1]'
  Selector : Selector  Elements=[1 2 3 6]  InputPortWidth=6
  thruster  allocation control1 : Subsystem  AncestorBlock=|
      | rov_design_analysis/ROV Controller
      | Design
      | Applications/1. Heading autopilot/thruster 
      | allocation control
  u : Outport
  wires:
  err/1 -> Selector/1
  Selector/1 -> thruster  allocation control1/1(vel)
  " input"/1 -> thruster  allocation control1/2(on/off)
  thruster  allocation control1/1(volt) -> u/1

== system P_decouple_single_rov/outer-loop  controller/P decoupled /inner-PI ==
  PI : Inport  Port=1  LatchInput=off
  Demux1 : Demux  Outputs=6
  Mux2 : Mux  Inputs=6
  P Controller2 : simulink_extras/Additional Linear/PID Controller  P=1  I=0  D=0
  P Controller4 : simulink_extras/Additional Linear/PID Controller  P=1  I=0  D=0
  PController1 : simulink_extras/Additional Linear/PID Controller  P=1  I=0  D=0
  PI Controller3 : simulink_extras/Additional Linear/PID Controller  P=1  I=0  D=0
  " " : Outport
  wires:
  PI Controller3/1 -> Mux2/3
  PController1/1 -> Mux2/1
  P Controller2/1 -> Mux2/2
  Demux1/1 -> PController1/1
  Demux1/2 -> P Controller2/1
  Demux1/3 -> PI Controller3/1
  Demux1/6 -> P Controller4/1
  P Controller4/1 -> Mux2/6
  PI/1 -> Demux1/1
  Mux2/1 -> " "/1

== system P_decouple_single_rov/pipeline  tracking planner  1/decoupled input/x25, y=0, z=50 yaw=1.57 ==
  Mux : Mux  Inputs=6
  Start : Constant  Value=15
  Start1 : Constant  Value=25
  Start2 : Constant  Value=1.57
  6 : Outport
  wires:
  Start1/1 -> Mux/1
  Mux/1 -> 6/1
  Start2/1 -> Mux/6
  Start/1 -> Mux/3

== system P_decouple_single_rov/pipeline  tracking planner  1/decoupled input/x=0,y=0, z=0 yaw=0   ==
  Mux : Mux  Inputs=6
  Start : Constant  Value=0
  Start1 : Constant  Value=0
  8 : Outport
  wires:
  Mux/1 -> 8/1
  Start1/1 -> Mux/1
  Start/1 -> Mux/3, Mux/2, Mux/6

== system P_decouple_single_rov/pipeline  tracking planner  1/decoupled input/x=15,y=0, z=45 yaw=0  ==
  Mux : Mux  Inputs=6
  Start1 : Constant  Value=15
  Start2 : Constant  Value=10
  Start3 : Constant  Value=0
  Start4 : Constant  Value=0
  3 : Outport
  wires:
  Mux/1 -> 3/1
  Start1/1 -> Mux/1
  Start2/1 -> Mux/3
  Start3/1 -> Mux/6
  Start4/1 -> Mux/2

== system P_decouple_single_rov/pipeline  tracking planner  1/decoupled input/x=25, z=45 yaw=0 ==
  Mux : Mux  Inputs=6
  Start : Constant  Value=10
  Start1 : Constant  Value=25
  Start2 : Constant  Value=0
  4 : Outport
  wires:
  Mux/1 -> 4/1
  Start1/1 -> Mux/1
  Start/1 -> Mux/3
  Start2/1 -> Mux/6

== system P_decouple_single_rov/pipeline  tracking planner  1/decoupled input/x=25,y=0, z=50 yaw=0 ==
  Mux : Mux  Inputs=6
  Start : Constant  Value=0
  Start1 : Constant  Value=25
  Start2 : Constant  Value=15
  5 : Outport
  wires:
  Start1/1 -> Mux/1
  Mux/1 -> 5/1
  Start/1 -> Mux/6
  Start2/1 -> Mux/3

== system P_decouple_single_rov/pipeline  tracking planner  1/decoupled input/x=25,y=40, z=50 yaw=0 ==
  Mux : Mux  Inputs=6
  Start : Constant  Value=0
  Start1 : Constant  Value=25
  Start2 : Constant  Value=15
  Start3 : Constant  Value=15
  7 : Outport
  wires:
  Start1/1 -> Mux/1
  Mux/1 -> 7/1
  Start/1 -> Mux/6
  Start2/1 -> Mux/2
  Start3/1 -> Mux/3

== system P_decouple_single_rov/pipeline  tracking planner  1/decoupled input/x=y=0, z=-50 yaw=0   ==
  Mux : Mux  Inputs=6
  Start : Constant  Value=15
  Start1 : Constant  Value=0
  Start2 : Constant  Value=0
  "1 " : Outport
  wires:
  Mux/1 -> "1 "/1
  Start1/1 -> Mux/1, Mux/2
  Start/1 -> Mux/3
  Start2/1 -> Mux/6

== system P_decouple_single_rov/pipeline  tracking planner  1/decoupled input/x=y=15, z=50 yaw=0  ==
  Mux : Mux  Inputs=6
  Start : Constant  Value=0
  Start1 : Constant  Value=15
  Start2 : Constant  Value=15
  2 : Outport
  wires:
  Mux/1 -> 2/1
  Start1/1 -> Mux/1
  Start2/1 -> Mux/3
  Start/1 -> Mux/6

== system P_decouple_single_rov/Thruster  Dynamic/thruster  dynamic     1/thruster  alloc. /thruster  allocation control1 ==
  vel : Inport  Orientation=down  Port=1  LatchInput=off
  on/off : Inport  Port=2  LatchInput=off
  "thruster allocation " : Subsystem
  volt : Outport
  wires:
  vel/1 -> "thruster allocation "/1(vel)
  on/off/1 -> "thruster allocation "/2(on/off)
  "thruster allocation "/1(volt) -> volt/1

== system P_decouple_single_rov/Thruster  Dynamic/thruster  dynamic     2/thruster  alloc. /thruster  allocation control1 ==
  vel : Inport  Orientation=down  Port=1  LatchInput=off
  on/off : Inport  Port=2  LatchInput=off
  "thruster allocation " : Subsystem
  volt : Outport
  wires:
  vel/1 -> "thruster allocation "/1(vel)
  on/off/1 -> "thruster allocation "/2(on/off)
  "thruster allocation "/1(volt) -> volt/1

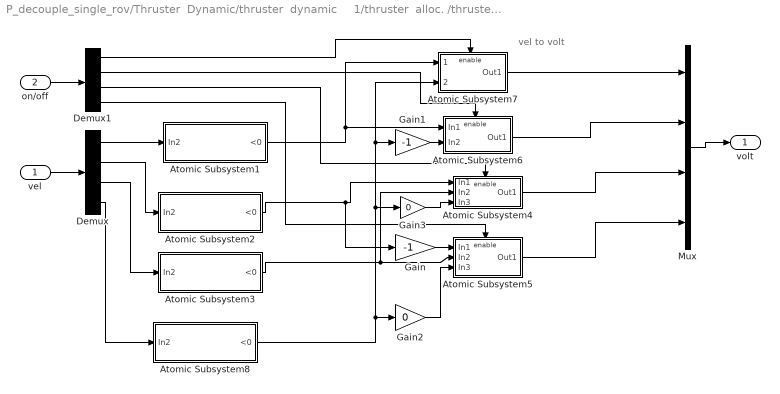
== system P_decouple_single_rov/Thruster  Dynamic/thruster  dynamic     1/thruster  alloc. /thruster  allocation control1/thruster allocation  ==
  note: vel to volt
  vel : Inport  Port=1  LatchInput=off
  on/off : Inport  Port=2  LatchInput=off
  Atomic Subsystem1 : Subsystem  TreatAsAtomicUnit=on
      mask Display: disp('check x >0, send \n signal to thrusters ')
  Atomic Subsystem2 : Subsystem  TreatAsAtomicUnit=on
      mask Display: disp('check y >0, send \n signal to thrusters ')
  Atomic Subsystem3 : Subsystem  TreatAsAtomicUnit=on
      mask Display: disp('check z >0, send \n signal to thrusters ')
  Atomic Subsystem4 : Subsystem  TreatAsAtomicUnit=on
      mask Display: disp('activate T3')
  Atomic Subsystem5 : Subsystem  TreatAsAtomicUnit=on
      mask Display: disp('activate T4')
  Atomic Subsystem6 : Subsystem  TreatAsAtomicUnit=on
      mask Display: disp('activate T2')
  Atomic Subsystem7 : Subsystem  TreatAsAtomicUnit=on
      mask Display: disp('activate T1')
  Atomic Subsystem8 : Subsystem  TreatAsAtomicUnit=on
      mask Display: disp('check yaw >0, send \n signal to thrusters ')
  Demux : Demux
  Demux1 : Demux
  Gain : Gain  Gain=-1
  Gain1 : Gain  Gain=-1
  Gain2 : Gain  Gain=0
  Gain3 : Gain  Gain=0
  Mux : Mux
  volt : Outport
  wires:
  Demux/1 -> Atomic Subsystem1/1(In2)
  Demux/2 -> Atomic Subsystem2/1(In2)
  Demux/3 -> Atomic Subsystem3/1(In2)
  Atomic Subsystem7/1(Out1) -> Mux/1
  vel/1 -> Demux/1
  Demux/4 -> Atomic Subsystem8/1(In2)
  on/off/1 -> Demux1/1
  Mux/1 -> volt/1
  Atomic Subsystem6/1(Out1) -> Mux/2
  Atomic Subsystem4/1(Out1) -> Mux/3
  Atomic Subsystem5/1(Out1) -> Mux/4
  Atomic Subsystem1/1(<0) -> Atomic Subsystem7/1(1), Atomic Subsystem6/1(In1)
  Atomic Subsystem2/1(<0) -> Atomic Subsystem4/1(In1), Gain/1
  Atomic Subsystem3/1(<0) -> Atomic Subsystem4/2(In2), Atomic Subsystem5/2(In2)
  Gain/1 -> Atomic Subsystem5/1(In1)
  Atomic Subsystem8/1(<0) -> Atomic Subsystem7/2(2), Gain1/1, Gain3/1, Gain2/1
  Gain1/1 -> Atomic Subsystem6/2(In2)
  Gain2/1 -> Atomic Subsystem5/3(In3)
  Demux1/1 -> Atomic Subsystem7/Enable
  Demux1/2 -> Atomic Subsystem6/Enable
  Demux1/3 -> Atomic Subsystem4/Enable
  Demux1/4 -> Atomic Subsystem5/Enable
  Gain3/1 -> Atomic Subsystem4/3(In3)
